simulink model "Report_capture"  (R2025a)
settings: Solver=VariableStepAuto  StartTime=0.0  StopTime=10.0  RelTol=1e-3
values from neighbouring files (symbols this model uses):
  b = 77.581e-6    (= 7.7581e-05)    [Lab2_params_student.m]    (also in P_controller_Calculate.m = 2*zeta*wn)
  J = 58.559e-6    (= 5.8559e-05)    [Lab2_params_student.m]
  L = 0.1    [Lab2_params_student.m]
  Lm = 2.8445e-3    (= 0.0028445)    [Lab2_params_student.m]
  mp = 0.05    [Lab2_params_student.m]
  R = 3.18    [Lab2_params_student.m]
undefined symbols (not defined in the file or in its folder): Eff, Ke, Km
settings Model: Creator=nitic  LastModifiedBy=nitic

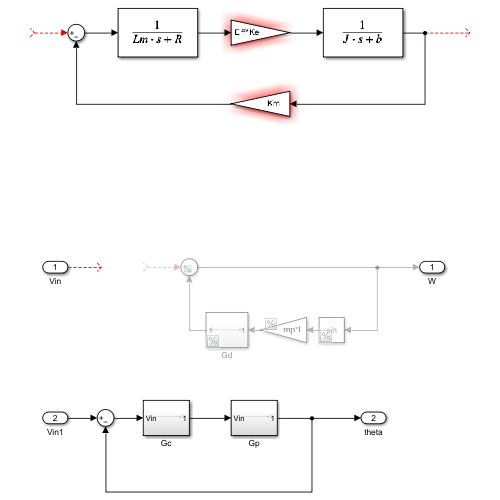
[thumbnail: Simulink's stored preview of the top-level diagram]
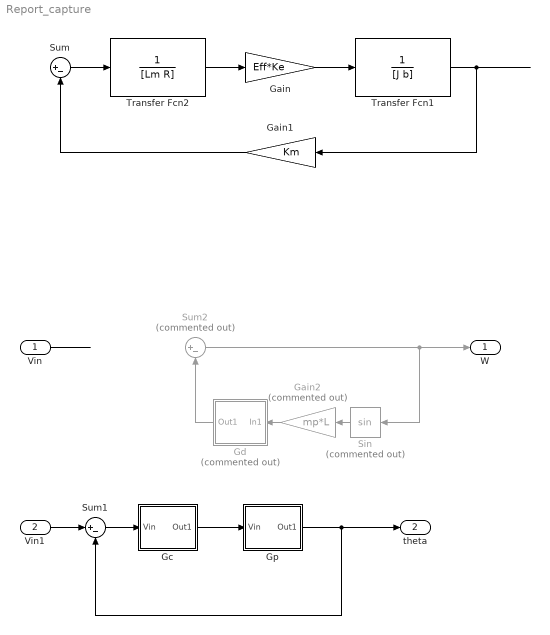
== system Report_capture ==
  Vin : Inport
  Vin1 : Inport  Port=2
  Gain : Gain  Gain=Eff*Ke
  Gain1 : Gain  Gain=Km
  Gain2 : Gain  Commented=on  Gain=mp*L
  Gc : Subsystem
  Gd : Subsystem  Commented=on
  Gp : Subsystem
  Sin : Trigonometry  Commented=on
  Sum : Sum  Inputs=|+-
  Sum1 : Sum  Inputs=|+-
  Sum2 : Sum  Commented=on  Inputs=|+-
  Transfer Fcn1 : TransferFcn  Denominator=[J b]
  Transfer Fcn2 : TransferFcn  Denominator=[Lm R]
  W : Outport
  theta : Outport  Port=2
  wires:
  ? -> Sum/1
  Sum/1 -> Transfer Fcn2/1
  Transfer Fcn2/1 -> Gain/1
  Gain/1 -> Transfer Fcn1/1
  Transfer Fcn1/1 -> Gain1/1
  Gain1/1 -> Sum/2
  Vin/1 -> ?
  Gain2/1 -> Gd/1(In1)
  Sin/1 -> Gain2/1
  Gd/1(Out1) -> Sum2/2
  ? -> Sum2/1
  Sum2/1 -> Sin/1, W/1
  Gp/1(Out1) -> theta/1, Sum1/2
  Gc/1(Out1) -> Gp/1(Vin)
  Vin1/1 -> Sum1/1
  Sum1/1 -> Gc/1(Vin)

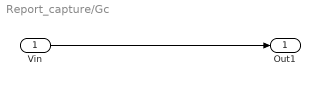
== system Report_capture/Gc ==
  Vin : Inport
  Out1 : Outport
  wires:
  Vin/1 -> Out1/1

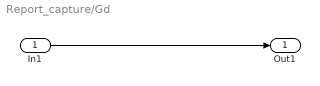
== system Report_capture/Gd ==
  In1 : Inport
  Out1 : Outport
  wires:
  In1/1 -> Out1/1

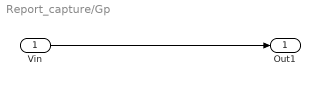
== system Report_capture/Gp ==
  Vin : Inport
  Out1 : Outport
  wires:
  Vin/1 -> Out1/1
